simulink model "ControleCartesiano"  (R2016a)
settings: Solver=VariableStepAuto  StartTime=0.0  StopTime=10.0  RelTol=1e-3
settings Model: Creator=User  LastModifiedBy=User

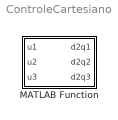
== system ControleCartesiano ==
  MATLAB Function : MATLAB Function  TreatAsAtomicUnit=on

== matlab function ControleCartesiano/MATLAB Function ==
  data: u1 input; d2q1 output; u2 input; u3 input; d2q2 output; d2q3 output
function [d2q1, d2q2, d2q3]= Sys(u1, u2, u3)

%%  Inicializações
u = [u1; u2; u3];
d2q = zeros(3,1);

%Parâmetros do sistema
Dinv = [ 0.0250     0           0
         0          0.0417      0
         0          0           0.1250];

G = [392.4000
     0
     0];
 
d2q = Dinv*(u-G);

d2q1 = d2q(1);
d2q2 = d2q(2);
d2q3 = d2q(3);
